simulink model "ITsystemThesis"  (R2025a)
settings: Solver=FixedStepAuto  StartTime=0.0  StopTime=0.55  FixedStep=50e-6  RelTol=1e-3
undefined symbols (not defined in the file): D1, Delta
libraries: spsSeriesRLCLoadLib x15, spsThreePhaseSeriesRLCLoadLib x12, spsPiSectionLineLib x12, spsThreePhasePISectionLineLib x11, spsThreePhaseVIMeasurementLib x7, spsThreePhaseTransformerTwoWindingsLib x6, spsSequenceAnalyzerLib x6, spsMultimeterLib x4, spsThreePhaseFaultLib x3, spsVoltageMeasurementLib x3, spsGroundLib x2, spsThreePhaseSourceLib x1
settings Model: Creator=baofengbaofeng  LastModifiedBy=baofeng
settings ModelReferenceCC: EnableRefExpFcnMdlSchedulingChecks=on
settings RTWCC: GPUComputeCapability=3.5  DLArmComputeVersion=19.05

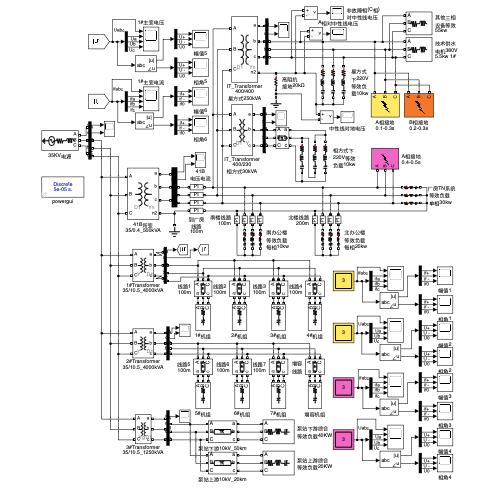
[thumbnail: Simulink's stored preview of the top-level diagram]
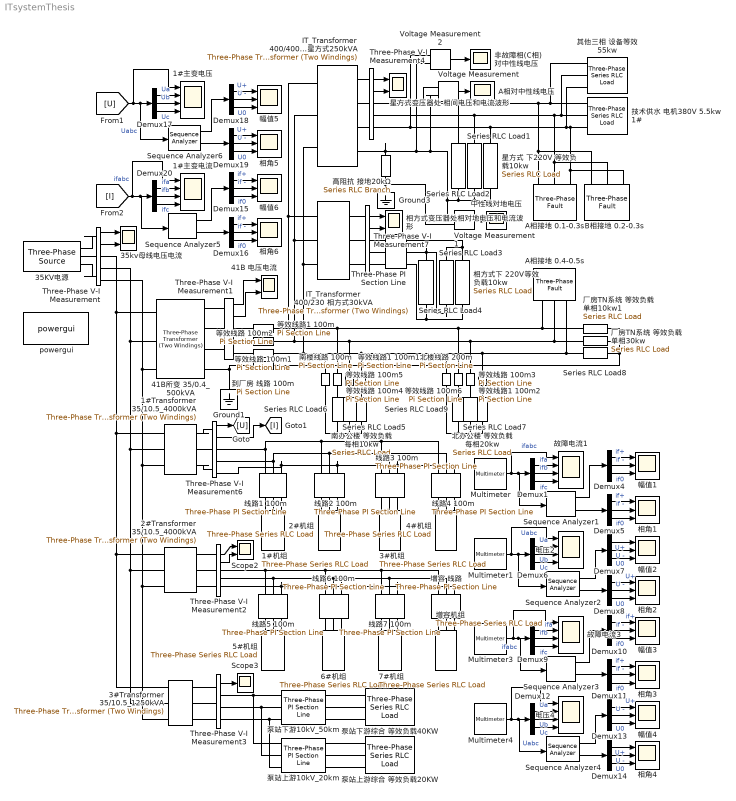
== system ITsystemThesis ==
  "    厂房TN系统 等效负载 单相10kw1" : spsSeriesRLCLoadLib/Series RLC Load  LConnTagsString=a  RConnTagsString=__new0  NominalVoltage=230  NominalFrequency=50  ActivePower=10e3  InductivePower=100  CapacitivePower=100  Setx0=off  InitialVoltage=0  SetiL0=off  InitialCurrent=0  Measurements=None  LoadType=constant Z
  "    厂房TN系统 等效负载 单相30kw" : spsSeriesRLCLoadLib/Series RLC Load  LConnTagsString=a  RConnTagsString=__new0  NominalVoltage=230  NominalFrequency=50  ActivePower=10e3  InductivePower=100  CapacitivePower=100  Setx0=off  InitialVoltage=0  SetiL0=off  InitialCurrent=0  Measurements=None  LoadType=constant Z
  1#Transformer 35/10.5_4000kVA : spsThreePhaseTransformerTwoWindingsLib/Three-Phase Transformer (Two Windings)  Winding1Connection=Y  Winding2Connection=Delta (D1)  CoreType=Three single-phase transformers  SetSaturation=off  Hysteresis=off  DataFile='hysteresis'  SetInitialFlux=off  Measurements=None  UNITS=pu  NominalPower=[4e6 , 50 ]  Winding1=[35000 0.01 0.049999]  Winding2=[10.5e3 0.01 0.05]  Rm=500  Lm=500  L0=0.5  Saturation=[0 0;0.0024 1.2;0.99998 1.52]  InitialFluxes=[ 0.8 , -0.8 , 0.7 ]  BreakLoop=off  DiscreteSolver=Trapezoidal iterative  DataType=off  TransfoNumber=1
  1#主变电压 : Scope  NumInputPorts=4
      settings: ActiveDisplayYMinimum=-10885.8844835699  ActiveDisplayYMaximum=10885.75905010345
  1#主变电流 : Scope  NumInputPorts=4
      settings: ActiveDisplayYMinimum=-290.20750490903231  ActiveDisplayYMaximum=290.20954287182195
  1#机组 : spsThreePhaseSeriesRLCLoadLib/Three-Phase Series RLC Load  LConnTagsString=A|B|C  Configuration=Delta  NominalVoltage=10e3  Vabc=[1e3 1e3 1e3]  Vabcp=[1e3 1e3 1e3]  NominalFrequency=50  UnbalancedPower=off  ActivePower=600e3  InductivePower=0  CapacitivePower=290e3  Pabc=[10e3 9e3 11e3]  QLabc=[100 90 110]  QCabc=[100 90 110]  Pabcp=[10e3 9e3 11e3]  QLabcp=[100 90 110]  QCabcp=[100 90 110]  Measurements=None  LoadType=constant PQ
  2#Transformer 35/10.5_4000kVA : spsThreePhaseTransformerTwoWindingsLib/Three-Phase Transformer (Two Windings)  Winding1Connection=Y  Winding2Connection=Delta (D1)  CoreType=Three single-phase transformers  SetSaturation=off  Hysteresis=off  DataFile='hysteresis'  SetInitialFlux=off  Measurements=None  UNITS=pu  NominalPower=[4e6 , 50 ]  Winding1=[35000 0.01 0.049999]  Winding2=[10.5e3 0.01 0.05]  Rm=500  Lm=500  L0=0.5  Saturation=[0 0;0.0024 1.2;0.99998 1.52]  InitialFluxes=[ 0.8 , -0.8 , 0.7 ]  BreakLoop=off  DiscreteSolver=Trapezoidal iterative  DataType=off  TransfoNumber=1
  2#机组 : spsThreePhaseSeriesRLCLoadLib/Three-Phase Series RLC Load  LConnTagsString=A|B|C  Configuration=Delta  NominalVoltage=10e3  Vabc=[1e3 1e3 1e3]  Vabcp=[1e3 1e3 1e3]  NominalFrequency=50  UnbalancedPower=off  ActivePower=600e3  InductivePower=0  CapacitivePower=290e3  Pabc=[10e3 9e3 11e3]  QLabc=[100 90 110]  QCabc=[100 90 110]  Pabcp=[10e3 9e3 11e3]  QLabcp=[100 90 110]  QCabcp=[100 90 110]  Measurements=None  LoadType=constant PQ
  3#Transformer 35/10.5_1250kVA : spsThreePhaseTransformerTwoWindingsLib/Three-Phase Transformer (Two Windings)  Winding1Connection=Yg  Winding2Connection=Delta (D1)  CoreType=Three single-phase transformers  SetSaturation=off  Hysteresis=off  DataFile='hysteresis'  SetInitialFlux=off  Measurements=None  UNITS=pu  NominalPower=[1250e3 , 50 ]  Winding1=[35000 0.01 0.049999]  Winding2=[10.5e3 0.01 0.05]  Rm=500  Lm=500  L0=0.5  Saturation=[0 0;0.0024 1.2;0.99998 1.52]  InitialFluxes=[ 0.8 , -0.8 , 0.7 ]  BreakLoop=off  DiscreteSolver=Trapezoidal iterative  DataType=off  TransfoNumber=1
  3#机组 : spsThreePhaseSeriesRLCLoadLib/Three-Phase Series RLC Load  LConnTagsString=A|B|C  Configuration=Delta  NominalVoltage=10e3  Vabc=[1e3 1e3 1e3]  Vabcp=[1e3 1e3 1e3]  NominalFrequency=50  UnbalancedPower=off  ActivePower=600e3  InductivePower=0  CapacitivePower=290e3  Pabc=[10e3 9e3 11e3]  QLabc=[100 90 110]  QCabc=[100 90 110]  Pabcp=[10e3 9e3 11e3]  QLabcp=[100 90 110]  QCabcp=[100 90 110]  Measurements=None  LoadType=constant PQ
  35KV电源 : spsThreePhaseSourceLib/Three-Phase Source  InternalConnection=Yg  VoltagePhases=off  Voltage=35e3  PhaseAngle=0  Voltage_phases=[25e3 25e3 25e3]/sqrt(3)  PhaseAngles_phases=[0 -120 +120]  Frequency=50  NonIdealSource=on  SpecifyImpedance=off  Resistance=0.1  Inductance=0.1e-3  ShortCircuitLevel=100e6  BaseVoltage=35e3  XRratio=7  BusType=swing  Pref=10e3  Qref=0  Prefabc=[10e3, 10e3, 10e3]  Qrefabc=[0, 0, 0]  Qmin=-inf  Qmax=inf
  35kv母线电压电流 : Scope  NumInputPorts=2
      settings: ActiveDisplayYMinimum=-35706.846494267083  ActiveDisplayYMaximum=35707.041687054967  DataLoggingVariableName=ScopeData6
  4#机组 : spsThreePhaseSeriesRLCLoadLib/Three-Phase Series RLC Load  LConnTagsString=A|B|C  Configuration=Delta  NominalVoltage=10e3  Vabc=[1e3 1e3 1e3]  Vabcp=[1e3 1e3 1e3]  NominalFrequency=50  UnbalancedPower=off  ActivePower=600e3  InductivePower=0  CapacitivePower=290e3  Pabc=[10e3 9e3 11e3]  QLabc=[100 90 110]  QCabc=[100 90 110]  Pabcp=[10e3 9e3 11e3]  QLabcp=[100 90 110]  QCabcp=[100 90 110]  Measurements=None  LoadType=constant PQ
  41B 电压电流 : Scope  NumInputPorts=2
      settings: ActiveDisplayYMinimum=-693.505234778138  ActiveDisplayYMaximum=693.42851734573628  DataLoggingVariableName=ScopeData2
  41B所变 35/0.4_500kVA : spsThreePhaseTransformerTwoWindingsLib/Three-Phase Transformer (Two Windings)  Winding1Connection=Delta (D1)  Winding2Connection=Yn  CoreType=Three single-phase transformers  SetSaturation=off  Hysteresis=off  DataFile='hysteresis'  SetInitialFlux=off  Measurements=None  UNITS=pu  NominalPower=[500e3 , 50 ]  Winding1=[35000 0.01 0.049999]  Winding2=[400 0.01 0.05]  Rm=500  Lm=499.99  L0=0.5  Saturation=[0 0;0.0024 1.2;0.99998 1.52]  InitialFluxes=[ 0.8 , -0.8 , 0.7 ]  BreakLoop=off  DiscreteSolver=Trapezoidal iterative  DataType=off  TransfoNumber=1
  5#机组 : spsThreePhaseSeriesRLCLoadLib/Three-Phase Series RLC Load  LConnTagsString=A|B|C  Configuration=Y (floating)  NominalVoltage=10e3  Vabc=[1e3 1e3 1e3]  Vabcp=[1e3 1e3 1e3]  NominalFrequency=50  UnbalancedPower=off  ActivePower=600e3  InductivePower=0  CapacitivePower=290e3  Pabc=[10e3 9e3 11e3]  QLabc=[100 90 110]  QCabc=[100 90 110]  Pabcp=[10e3 9e3 11e3]  QLabcp=[100 90 110]  QCabcp=[100 90 110]  Measurements=None  LoadType=constant PQ
  6#机组 : spsThreePhaseSeriesRLCLoadLib/Three-Phase Series RLC Load  LConnTagsString=A|B|C  Configuration=Y (floating)  NominalVoltage=10e3  Vabc=[1e3 1e3 1e3]  Vabcp=[1e3 1e3 1e3]  NominalFrequency=50  UnbalancedPower=off  ActivePower=600e3  InductivePower=0  CapacitivePower=290e3  Pabc=[10e3 9e3 11e3]  QLabc=[100 90 110]  QCabc=[100 90 110]  Pabcp=[10e3 9e3 11e3]  QLabcp=[100 90 110]  QCabcp=[100 90 110]  Measurements=None  LoadType=constant PQ
  7#机组 : spsThreePhaseSeriesRLCLoadLib/Three-Phase Series RLC Load  LConnTagsString=A|B|C  Configuration=Y (floating)  NominalVoltage=10e3  Vabc=[1e3 1e3 1e3]  Vabcp=[1e3 1e3 1e3]  NominalFrequency=50  UnbalancedPower=off  ActivePower=600e3  InductivePower=0  CapacitivePower=290e3  Pabc=[10e3 9e3 11e3]  QLabc=[100 90 110]  QCabc=[100 90 110]  Pabcp=[10e3 9e3 11e3]  QLabcp=[100 90 110]  QCabcp=[100 90 110]  Measurements=None  LoadType=constant PQ
  A相对中性线电压 : Scope
      settings: ActiveDisplayYMinimum=-1  ActiveDisplayYMaximum=1  DataLoggingVariableName=ScopeData7
  A相接地 0.1-0.3s : spsThreePhaseFaultLib/Three-Phase Fault  InitialStates=0  FaultA=on  FaultB=off  FaultC=off  GroundFault=on  SwitchTimes="[5/50  15/50]"  External=off  SwitchStatus=NaN  FaultResistance=0.001  GroundResistance=0.01  SnubberResistance=20e3  SnubberCapacitance=1  Measurements=Fault voltages and currents
  A相接地 0.4-0.5s : spsThreePhaseFaultLib/Three-Phase Fault  InitialStates=0  FaultA=on  FaultB=off  FaultC=off  GroundFault=on  SwitchTimes="[20/50  25/50]"  External=off  SwitchStatus=NaN  FaultResistance=0.001  GroundResistance=0.01  SnubberResistance=1e3  SnubberCapacitance=inf  Measurements=Fault voltages and currents
  B相接地 0.2-0.3s : spsThreePhaseFaultLib/Three-Phase Fault  InitialStates=0  FaultA=off  FaultB=on  FaultC=off  GroundFault=on  SwitchTimes="[10/50  15/50]"  External=off  SwitchStatus=NaN  FaultResistance=0.001  GroundResistance=0.01  SnubberResistance=20e3  SnubberCapacitance=inf  Measurements=Fault voltages and currents
  Demux{1,4..20} (18 alike) : Demux  Outputs=3
  Ground1 : spsGroundLib/Ground  LConnTagsString=a
  Ground3 : spsGroundLib/Ground  LConnTagsString=a
  IT_Transformer 400/230 相方式30kVA : spsThreePhaseTransformerTwoWindingsLib/Three-Phase Transformer (Two Windings)  Winding1Connection=Delta (D1)  Winding2Connection=Y  CoreType=Three single-phase transformers  SetSaturation=off  Hysteresis=off  DataFile='hysteresis'  SetInitialFlux=off  Measurements=None  UNITS=pu  NominalPower=[30e3 , 50 ]  Winding1=[400, 0.002 , 0.08 ]  Winding2=[230, 0.002 , 0.08 ]  Rm=500  Lm=500  L0=0.5  Saturation=[ 0,0 ; 0.0024,1.2 ; 1.0,1.52 ]  InitialFluxes=[ 0.8 , -0.8 , 0.7 ]  BreakLoop=off  DiscreteSolver=Trapezoidal iterative  DataType=off  TransfoNumber=1
  IT_Transformer 400/400 星方式250kVA : spsThreePhaseTransformerTwoWindingsLib/Three-Phase Transformer (Two Windings)  Winding1Connection=Delta (D1)  Winding2Connection=Yn  CoreType=Three single-phase transformers  SetSaturation=off  Hysteresis=off  DataFile='hysteresis'  SetInitialFlux=off  Measurements=None  UNITS=pu  NominalPower=[ 250e3 , 50 ]  Winding1=[ 400 , 0.002 , 0.08 ]  Winding2=[ 400 , 0.002 , 0.08 ]  Rm=500  Lm=500  L0=0.5  Saturation=[ 0,0 ; 0.0024,1.2 ; 1.0,1.52 ]  InitialFluxes=[ 0.8 , -0.8 , 0.7 ]  BreakLoop=off  DiscreteSolver=Trapezoidal iterative  DataType=off  TransfoNumber=1
  Multimeter : spsMultimeterLib/Multimeter  L=12  sel=[7 8 9]  yselected={}  Gain=[1 1 1]  OutputType=Complex  PlotAtSimulationStop=off  PhasorSimulation=off
  Multimeter1 : spsMultimeterLib/Multimeter  L=12  sel=[1 2 3]  yselected={}  Gain=[1 1 1]  OutputType=Complex  PlotAtSimulationStop=off  PhasorSimulation=off
  Multimeter3 : spsMultimeterLib/Multimeter  L=12  sel=[10 11 12]  yselected={}  Gain=[1 1 1]  OutputType=Complex  PlotAtSimulationStop=off  PhasorSimulation=off
  Multimeter4 : spsMultimeterLib/Multimeter  L=12  sel=[4 5 6]  yselected={}  Gain=[1 1 1]  OutputType=Complex  PlotAtSimulationStop=off  PhasorSimulation=off
  Scope2 : Scope  NumInputPorts=2
      settings: ActiveDisplayYMinimum=-10885.884483600445  ActiveDisplayYMaximum=10885.759050087665  DataLoggingVariableName=ScopeData4
  Scope3 : Scope
      settings: ActiveDisplayYMinimum=-10727.159391884898  ActiveDisplayYMaximum=10726.597579018544  DataLoggingVariableName=ScopeData5
  Sequence Analyzer{1..6} (6 alike) : spsSequenceAnalyzerLib/Sequence Analyzer  Freq=50  n=1  seq=Positive Negative Zero  InInit=[1, 0]  Ts=0
      settings: LibrarySourceBlock=sps_lib/Sensors and Measurements/Sequence Analyzer
  Series RLC Load{1..6,8} (7 alike) : spsSeriesRLCLoadLib/Series RLC Load  LConnTagsString=a  RConnTagsString=__new0  NominalVoltage=230  NominalFrequency=50  ActivePower=10e3  InductivePower=100  CapacitivePower=100  Setx0=off  InitialVoltage=0  SetiL0=off  InitialCurrent=0  Measurements=None  LoadType=constant Z
  Series RLC Load7 : spsSeriesRLCLoadLib/Series RLC Load  LConnTagsString=a  RConnTagsString=__new0  NominalVoltage=230  NominalFrequency=50  ActivePower=20e3  InductivePower=100  CapacitivePower=100  Setx0=off  InitialVoltage=0  SetiL0=off  InitialCurrent=0  Measurements=None  LoadType=constant Z
  Series RLC Load9 : spsSeriesRLCLoadLib/Series RLC Load  LConnTagsString=a  RConnTagsString=__new0  NominalVoltage=230  NominalFrequency=50  ActivePower=20e3  InductivePower=100  CapacitivePower=100  Setx0=off  InitialVoltage=0  SetiL0=off  InitialCurrent=0  Measurements=None  LoadType=constant Z
  Three-Phase PI Section Line : spsThreePhasePISectionLineLib/Three-Phase PI Section Line  LConnTagsString=a|b|c  RConnTagsString=A|B|C  Length=100  Frequency=60  Resistances=[ 0.01273 0.3864]  Inductances="[ 0.9337e-3  4.1264e-3]"  Capacitances=[12.74e-9 7.751e-9]
  Three-Phase V-I Measurement{,2,6..7} (4 alike) : spsThreePhaseVIMeasurementLib/Three-Phase V-I Measurement  VoltageMeasurement=phase-to-ground  SetLabelV=off  LabelV=Vabc  Vpu=off  VpuLL=off  CurrentMeasurement=yes  SetLabelI=off  LabelI=Iabc  Ipu=off  Pbase=100e6  Vbase=500e3  OutputType=Complex  PhasorSimulation=off  PSBequivalent=0
  Three-Phase V-I Measurement1 : spsThreePhaseVIMeasurementLib/Three-Phase V-I Measurement  VoltageMeasurement=phase-to-phase  SetLabelV=off  LabelV=Vabc  Vpu=off  VpuLL=off  CurrentMeasurement=yes  SetLabelI=off  LabelI=Iabc  Ipu=off  Pbase=100e6  Vbase=500e3  OutputType=Complex  PhasorSimulation=off  PSBequivalent=0
  Three-Phase V-I Measurement3 : spsThreePhaseVIMeasurementLib/Three-Phase V-I Measurement  VoltageMeasurement=phase-to-ground  SetLabelV=off  LabelV=Vabc  Vpu=off  VpuLL=off  CurrentMeasurement=no  SetLabelI=off  LabelI=Iabc  Ipu=off  Pbase=100e6  Vbase=500e3  OutputType=Complex  PhasorSimulation=off  PSBequivalent=0
  Three-Phase V-I Measurement4 : spsThreePhaseVIMeasurementLib/Three-Phase V-I Measurement  VoltageMeasurement=phase-to-phase  SetLabelV=off  LabelV=Vabc  Vpu=off  VpuLL=off  CurrentMeasurement=yes  SetLabelI=off  LabelI=Iabc  Ipu=off  Pbase=100e6  Vbase=500e3  OutputType=Complex  PhasorSimulation=off  PSBequivalent=0
  Voltage Measurement : spsVoltageMeasurementLib/Voltage Measurement  PhasorSimulation=off  OutputType=Complex  PSBequivalent=0
  Voltage Measurement1 : spsVoltageMeasurementLib/Voltage Measurement  PhasorSimulation=off  OutputType=Complex  PSBequivalent=0
  Voltage Measurement2 : spsVoltageMeasurementLib/Voltage Measurement  PhasorSimulation=off  OutputType=Complex  PSBequivalent=0
  powergui : spspowerguiLib/powergui  Priority=1  SimulationMode=Discrete  SampleTime=50e-6  frequency=50  Iterations=50  frequencyindice=50  Pbase=100e6  ErrMax=1e-4  UnitsV=kV  UnitsW=MW  buscounter=0  FunctionMessages=off  echomessages=off  EnableUseOfTLC=off  CurrentSourceSwitches=off  DisableSnubberDevices=off  DisableRonSwitches=off  DisableVfSwitches=off  DisplayEquations=off  AutomaticDiscreteSolvers=off  SolverType=Tustin/Backward Euler (TBE)  Interpol=off  ExternalGateDelay=off  methode=off  Ts=100  x0status=blocks  SPID=on  SwTol=0  HookPort=off  NonlinearTolerance=1e-4  nMaxIteration=100  ContinueOnMaxIteration=off  RestoreLinks=warning  ResistiveCurrentMeasurement=off  Frange=[0:2:500]  Ylog=off  Xlog=on  ShowGrid=off  save=off  variable=ZData  structure=0  ZoomFFT=off  StartTime=0.0  cycles=1  DisplayStyle=1  fundamental=60  FreqAxis=off  MaxFrequency=1000  frequencyindicesteady=1  RmsSteady=1  display=off
  中性线对地电压 : Scope
      settings: ActiveDisplayYMinimum=-386.53820546977795  ActiveDisplayYMaximum=386.53827874690307  DataLoggingVariableName=ScopeData8
  其他三相 设备等效 55kw : spsThreePhaseSeriesRLCLoadLib/Three-Phase Series RLC Load  LConnTagsString=A|B|C  Configuration=Y (floating)  NominalVoltage=380  Vabc=[1e3 1e3 1e3]  Vabcp=[1e3 1e3 1e3]  NominalFrequency=50  UnbalancedPower=off  ActivePower=55e3  InductivePower=27.5e3  CapacitivePower=0  Pabc=[10e3 9e3 11e3]  QLabc=[100 90 110]  QCabc=[100 90 110]  Pabcp=[10e3 9e3 11e3]  QLabcp=[100 90 110]  QCabcp=[100 90 110]  Measurements=None  LoadType=constant Z
  到厂房 线路 100m : spsPiSectionLineLib/Pi Section Line  LConnTagsString=1  RConnTagsString=1  Phases=1  PiSections=1  Length=0.1  Frequency=50  Resistance=0.01273  Inductance=0.9337e-3  Capacitance=12.74e-9  SpecifyConductance=off  Conductance=0  Measurements=None  Measurements2=None
      settings: LibrarySourceBlock=sps_lib/Power Grid Elements/Pi Section Line
  北办公楼 等效负载 每相20kw : spsSeriesRLCLoadLib/Series RLC Load  LConnTagsString=a  RConnTagsString=__new0  NominalVoltage=230  NominalFrequency=50  ActivePower=20e3  InductivePower=100  CapacitivePower=100  Setx0=off  InitialVoltage=0  SetiL0=off  InitialCurrent=0  Measurements=None  LoadType=constant Z
  北楼线路 200m : spsPiSectionLineLib/Pi Section Line  LConnTagsString=1  RConnTagsString=1  Phases=1  PiSections=1  Length=0.2  Frequency=50  Resistance=0.01273  Inductance=0.9337e-3  Capacitance=12.74e-9  SpecifyConductance=off  Conductance=0  Measurements=None  Measurements2=None
      settings: LibrarySourceBlock=sps_lib/Power Grid Elements/Pi Section Line
  南办公楼 等效负载 每相10kw : spsSeriesRLCLoadLib/Series RLC Load  LConnTagsString=a  RConnTagsString=__new0  NominalVoltage=230  NominalFrequency=50  ActivePower=10e3  InductivePower=100  CapacitivePower=100  Setx0=off  InitialVoltage=0  SetiL0=off  InitialCurrent=0  Measurements=None  LoadType=constant Z
  南楼线路 100m : spsPiSectionLineLib/Pi Section Line  LConnTagsString=1  RConnTagsString=1  Phases=1  PiSections=1  Length=0.1  Frequency=50  Resistance=0.01273  Inductance=0.9337e-3  Capacitance=12.74e-9  SpecifyConductance=off  Conductance=0  Measurements=None  Measurements2=None
      settings: LibrarySourceBlock=sps_lib/Power Grid Elements/Pi Section Line
  增容 线路 : spsThreePhasePISectionLineLib/Three-Phase PI Section Line  LConnTagsString=a|b|c  RConnTagsString=A|B|C  Length=0.1  Frequency=50  Resistances=[ 0.01273 0.3864]  Inductances="[ 0.9337e-3  4.1264e-3]"  Capacitances=[12.74e-9 7.751e-9]
  增容机组 : spsThreePhaseSeriesRLCLoadLib/Three-Phase Series RLC Load  LConnTagsString=A|B|C  Configuration=Y (floating)  NominalVoltage=10e3  Vabc=[1e3 1e3 1e3]  Vabcp=[1e3 1e3 1e3]  NominalFrequency=50  UnbalancedPower=off  ActivePower=600e3  InductivePower=0  CapacitivePower=290e3  Pabc=[10e3 9e3 11e3]  QLabc=[100 90 110]  QCabc=[100 90 110]  Pabcp=[10e3 9e3 11e3]  QLabcp=[100 90 110]  QCabcp=[100 90 110]  Measurements=None  LoadType=constant PQ
  幅值{1..6} (6 alike) : Scope  NumInputPorts=3
      幅值1 settings: ActiveDisplayYMinimum=-0.00269711612383589  ActiveDisplayYMaximum=0.024274045114523017  DataLoggingVariableName=ScopeData11
      幅值2 settings: ActiveDisplayYMinimum=-37.543097825269918  ActiveDisplayYMaximum=347.88788042742931  DataLoggingVariableName=ScopeData14
      幅值3 settings: ActiveDisplayYMinimum=-237.57858107654377  ActiveDisplayYMaximum=2138.2072296888946  DataLoggingVariableName=ScopeData19
      幅值4 settings: ActiveDisplayYMinimum=-39.338118269801356  ActiveDisplayYMaximum=364.04306442821229  DataLoggingVariableName=ScopeData20
      幅值5 settings: ActiveDisplayYMinimum=-1087.411711387326  ActiveDisplayYMaximum=9796.7054024859353  DataLoggingVariableName=ScopeData24
      幅值6 settings: ActiveDisplayYMinimum=-27.894504137772689  ActiveDisplayYMaximum=261.05053723995428  DataLoggingVariableName=ScopeData23
  技术供水 电机380V 5.5kw 1# : spsThreePhaseSeriesRLCLoadLib/Three-Phase Series RLC Load  LConnTagsString=A|B|C  Configuration=Y (floating)  NominalVoltage=380  Vabc=[1e3 1e3 1e3]  Vabcp=[1e3 1e3 1e3]  NominalFrequency=50  UnbalancedPower=off  ActivePower=5.5e3  InductivePower=2.75e3  CapacitivePower=0  Pabc=[10e3 9e3 11e3]  QLabc=[100 90 110]  QCabc=[100 90 110]  Pabcp=[10e3 9e3 11e3]  QLabcp=[100 90 110]  QCabcp=[100 90 110]  Measurements=None  LoadType=constant Z
  故障电流1 : Scope  NumInputPorts=4
      settings: ActiveDisplayYMinimum=-2115.6411271895017  ActiveDisplayYMaximum=2117.5918585380573  DataLoggingVariableName=ScopeData3
  故障电流3 : Scope  NumInputPorts=4
      settings: ActiveDisplayYMinimum=-6472.8025751599744  ActiveDisplayYMaximum=8249.2362367472233  DataLoggingVariableName=ScopeData18
  星方式 下220V 等效负 载10kw : spsSeriesRLCLoadLib/Series RLC Load  LConnTagsString=a  RConnTagsString=__new0  NominalVoltage=230  NominalFrequency=50  ActivePower=10e3  InductivePower=100  CapacitivePower=100  Setx0=off  InitialVoltage=0  SetiL0=off  InitialCurrent=0  Measurements=None  LoadType=constant Z
  星方式变压器处 相间电压和电流波形 : Scope  NumInputPorts=2
      settings: ActiveDisplayYMinimum=-670.32665640027585  ActiveDisplayYMaximum=669.92281587607806  DataLoggingVariableName=ScopeData15
  泵站上游10kV_20km : spsThreePhasePISectionLineLib/Three-Phase PI Section Line  LConnTagsString=a|b|c  RConnTagsString=A|B|C  Length=20  Frequency=50  Resistances=[ 0.01273 0.3864]  Inductances="[ 0.9337e-3  4.1264e-3]"  Capacitances=[12.74e-9 7.751e-9]
  泵站上游综合 等效负载20KW : spsThreePhaseSeriesRLCLoadLib/Three-Phase Series RLC Load  LConnTagsString=A|B|C  Configuration=Y (floating)  NominalVoltage=10e3  Vabc=[1e3 1e3 1e3]  Vabcp=[1e3 1e3 1e3]  NominalFrequency=50  UnbalancedPower=off  ActivePower=20e3  InductivePower=100  CapacitivePower=100  Pabc=[10e3 9e3 11e3]  QLabc=[100 90 110]  QCabc=[100 90 110]  Pabcp=[10e3 9e3 11e3]  QLabcp=[100 90 110]  QCabcp=[100 90 110]  Measurements=None  LoadType=constant Z
  泵站下游10kV_50km : spsThreePhasePISectionLineLib/Three-Phase PI Section Line  LConnTagsString=a|b|c  RConnTagsString=A|B|C  Length=50  Frequency=50  Resistances=[ 0.01273 0.3864]  Inductances="[ 0.9337e-3  4.1264e-3]"  Capacitances=[12.74e-9 7.751e-9]
  泵站下游综合 等效负载40KW : spsThreePhaseSeriesRLCLoadLib/Three-Phase Series RLC Load  LConnTagsString=A|B|C  Configuration=Y (floating)  NominalVoltage=10e3  Vabc=[1e3 1e3 1e3]  Vabcp=[1e3 1e3 1e3]  NominalFrequency=50  UnbalancedPower=off  ActivePower=40e3  InductivePower=100  CapacitivePower=100  Pabc=[10e3 9e3 11e3]  QLabc=[100 90 110]  QCabc=[100 90 110]  Pabcp=[10e3 9e3 11e3]  QLabcp=[100 90 110]  QCabcp=[100 90 110]  Measurements=None  LoadType=constant Z
  电压2 : Scope  NumInputPorts=4
      settings: ActiveDisplayYMinimum=-669.7122622202794  ActiveDisplayYMaximum=669.712217692271  DataLoggingVariableName=ScopeData12
  电压4 : Scope  NumInputPorts=4
      settings: ActiveDisplayYMinimum=-475.45137271071371  ActiveDisplayYMaximum=457.036637182715  DataLoggingVariableName=ScopeData17
  相方式下 220V等效 负载10kw : spsSeriesRLCLoadLib/Series RLC Load  LConnTagsString=a  RConnTagsString=__new0  NominalVoltage=230  NominalFrequency=50  ActivePower=10e3  InductivePower=100  CapacitivePower=100  Setx0=off  InitialVoltage=0  SetiL0=off  InitialCurrent=0  Measurements=None  LoadType=constant Z
  相方式变压器处相对地电压和电流波形 : Scope  NumInputPorts=2
      settings: ActiveDisplayYMinimum=-229.68543143110043  ActiveDisplayYMaximum=227.02248165488766  DataLoggingVariableName=ScopeData16
  相角{1..6} (6 alike) : Scope  NumInputPorts=3
      相角1 settings: ActiveDisplayYMinimum=-1  ActiveDisplayYMaximum=1  DataLoggingVariableName=ScopeData10
      相角2 settings: ActiveDisplayYMinimum=-7.0496414728403192  ActiveDisplayYMaximum=63.446773255562888  DataLoggingVariableName=ScopeData13
      相角3 settings: ActiveDisplayYMinimum=-160.42500077107547  ActiveDisplayYMaximum=116.32499922893246  DataLoggingVariableName=ScopeData21
      相角4 settings: ActiveDisplayYMinimum=-3.4641360988234386  ActiveDisplayYMaximum=31.177224889410954  DataLoggingVariableName=ScopeData22
      相角5 settings: ActiveDisplayYMinimum=-39.040360895201125  ActiveDisplayYMaximum=4.3378178772445688  DataLoggingVariableName=ScopeData26
      相角6 settings: ActiveDisplayYMinimum=-1  ActiveDisplayYMaximum=1  DataLoggingVariableName=ScopeData25
  等效线路 100m{1..2,4..5} (4 alike) : spsPiSectionLineLib/Pi Section Line  LConnTagsString=1  RConnTagsString=1  Phases=1  PiSections=1  Length=0.1  Frequency=50  Resistance=0.01273  Inductance=0.9337e-3  Capacitance=12.74e-9  SpecifyConductance=off  Conductance=0  Measurements=None  Measurements2=None
      settings: LibrarySourceBlock=sps_lib/Power Grid Elements/Pi Section Line
  等效线路 100m3 : spsPiSectionLineLib/Pi Section Line  LConnTagsString=1  RConnTagsString=1  Phases=1  PiSections=1  Length=0.2  Frequency=50  Resistance=0.01273  Inductance=0.9337e-3  Capacitance=12.74e-9  SpecifyConductance=off  Conductance=0  Measurements=None  Measurements2=None
      settings: LibrarySourceBlock=sps_lib/Power Grid Elements/Pi Section Line
  等效线路 100m6 : spsPiSectionLineLib/Pi Section Line  LConnTagsString=1  RConnTagsString=1  Phases=1  PiSections=1  Length=0.2  Frequency=50  Resistance=0.01273  Inductance=0.9337e-3  Capacitance=12.74e-9  SpecifyConductance=off  Conductance=0  Measurements=None  Measurements2=None
      settings: LibrarySourceBlock=sps_lib/Power Grid Elements/Pi Section Line
  等效线路1 100m : spsPiSectionLineLib/Pi Section Line  LConnTagsString=1  RConnTagsString=1  Phases=1  PiSections=1  Length=0.1  Frequency=50  Resistance=0.01273  Inductance=0.9337e-3  Capacitance=12.74e-9  SpecifyConductance=off  Conductance=0  Measurements=None  Measurements2=None
      settings: LibrarySourceBlock=sps_lib/Power Grid Elements/Pi Section Line
  等效线路1 100m1 : spsPiSectionLineLib/Pi Section Line  LConnTagsString=1  RConnTagsString=1  Phases=1  PiSections=1  Length=0.1  Frequency=50  Resistance=0.01273  Inductance=0.9337e-3  Capacitance=12.74e-9  SpecifyConductance=off  Conductance=0  Measurements=None  Measurements2=None
      settings: LibrarySourceBlock=sps_lib/Power Grid Elements/Pi Section Line
  等效线路1 100m2 : spsPiSectionLineLib/Pi Section Line  LConnTagsString=1  RConnTagsString=1  Phases=1  PiSections=1  Length=0.2  Frequency=50  Resistance=0.01273  Inductance=0.9337e-3  Capacitance=12.74e-9  SpecifyConductance=off  Conductance=0  Measurements=None  Measurements2=None
      settings: LibrarySourceBlock=sps_lib/Power Grid Elements/Pi Section Line
  线路1 100m : spsThreePhasePISectionLineLib/Three-Phase PI Section Line  LConnTagsString=a|b|c  RConnTagsString=A|B|C  Length=0.1  Frequency=50  Resistances=[ 0.01273 0.3864]  Inductances="[ 0.9337e-3  4.1264e-3]"  Capacitances=[12.74e-9 7.751e-9]
  线路2 100m : spsThreePhasePISectionLineLib/Three-Phase PI Section Line  LConnTagsString=a|b|c  RConnTagsString=A|B|C  Length=0.1  Frequency=50  Resistances=[ 0.01273 0.3864]  Inductances="[ 0.9337e-3  4.1264e-3]"  Capacitances=[12.74e-9 7.751e-9]
  线路3 100m : spsThreePhasePISectionLineLib/Three-Phase PI Section Line  LConnTagsString=a|b|c  RConnTagsString=A|B|C  Length=0.1  Frequency=50  Resistances=[ 0.01273 0.3864]  Inductances="[ 0.9337e-3  4.1264e-3]"  Capacitances=[12.74e-9 7.751e-9]
  线路4 100m : spsThreePhasePISectionLineLib/Three-Phase PI Section Line  LConnTagsString=a|b|c  RConnTagsString=A|B|C  Length=0.1  Frequency=50  Resistances=[ 0.01273 0.3864]  Inductances="[ 0.9337e-3  4.1264e-3]"  Capacitances=[12.74e-9 7.751e-9]
  线路5 100m : spsThreePhasePISectionLineLib/Three-Phase PI Section Line  LConnTagsString=a|b|c  RConnTagsString=A|B|C  Length=0.1  Frequency=50  Resistances=[ 0.01273 0.3864]  Inductances="[ 0.9337e-3  4.1264e-3]"  Capacitances=[12.74e-9 7.751e-9]
  线路6 100m : spsThreePhasePISectionLineLib/Three-Phase PI Section Line  LConnTagsString=a|b|c  RConnTagsString=A|B|C  Length=0.1  Frequency=50  Resistances=[ 0.01273 0.3864]  Inductances="[ 0.9337e-3  4.1264e-3]"  Capacitances=[12.74e-9 7.751e-9]
  线路7 100m : spsThreePhasePISectionLineLib/Three-Phase PI Section Line  LConnTagsString=a|b|c  RConnTagsString=A|B|C  Length=0.1  Frequency=50  Resistances=[ 0.01273 0.3864]  Inductances="[ 0.9337e-3  4.1264e-3]"  Capacitances=[12.74e-9 7.751e-9]
  非故障相(C相) 对中性线电压 : Scope
      settings: ActiveDisplayYMinimum=-1  ActiveDisplayYMaximum=1  DataLoggingVariableName=ScopeData9
  高阻抗 接地20kΩ : spsSeriesRLCBranchLib/Series RLC Branch  LConnTagsString=__new0  RConnTagsString=__new0  BranchType=R  Resistance=20000  Inductance=0  SetiL0=off  InitialCurrent=0  Capacitance=0  Setx0=off  InitialVoltage=0  Measurements=None
  wires:
  Three-Phase V-I Measurement6/1 -> [U]
  Three-Phase V-I Measurement2/1 -> Scope2/1
  Three-Phase V-I Measurement/1 -> 35kv母线电压电流/1
  Three-Phase V-I Measurement3/1 -> Scope3/1
  Three-Phase V-I Measurement/2 -> 35kv母线电压电流/2
  Three-Phase V-I Measurement1/2 -> 41B 电压电流/2
  Three-Phase V-I Measurement2/2 -> Scope2/2
  Three-Phase V-I Measurement1/1 -> 41B 电压电流/1
  Demux5/3 -> 相角1/3  "if0"
  Demux1/3 -> 故障电流1/4  "ifc"
  Multimeter/1 -> Sequence Analyzer1/1, Demux1/1, 故障电流1/1  "ifabc"
  Demux5/1 -> 相角1/1  "if+"
  Demux5/2 -> 相角1/2  "if -"
  Demux1/1 -> 故障电流1/2  "ifa"
  Demux4/3 -> 幅值1/3  "if0"
  Demux1/2 -> 故障电流1/3  "ifb"
  Demux4/1 -> 幅值1/1  "if+"
  Demux4/2 -> 幅值1/2  "if -"
  Sequence Analyzer1/2 -> Demux5/1
  Sequence Analyzer1/1 -> Demux4/1
  Demux7/3 -> 幅值2/3  "U0"
  Demux8/2 -> 相角2/2  "U -"
  Demux6/2 -> 电压2/3  "Ub"
  Demux6/3 -> 电压2/4  "Uc"
  Sequence Analyzer2/2 -> Demux8/1
  Demux7/1 -> 幅值2/1  "U+"
  Demux8/3 -> 相角2/3  "U0"
  Demux8/1 -> 相角2/1  "U+"
  Demux7/2 -> 幅值2/2  "U -"
  Multimeter1/1 -> 电压2/1, Demux6/1, Sequence Analyzer2/1  "Uabc"
  Sequence Analyzer2/1 -> Demux7/1
  Three-Phase V-I Measurement4/1 -> 星方式变压器处 相间电压和电流波形/1
  Three-Phase V-I Measurement4/2 -> 星方式变压器处 相间电压和电流波形/2
  Three-Phase V-I Measurement7/1 -> 相方式变压器处相对地电压和电流波形/1
  Three-Phase V-I Measurement7/2 -> 相方式变压器处相对地电压和电流波形/2
  Demux6/1 -> 电压2/2  "Ua"
  Demux12/1 -> 电压4/2  "Ua"
  Sequence Analyzer4/1 -> Demux13/1
  Multimeter4/1 -> Sequence Analyzer4/1, Demux12/1, 电压4/1  "Uabc"
  Demux13/2 -> 幅值4/2  "U -"
  Demux14/1 -> 相角4/1  "U+"
  Demux14/3 -> 相角4/3  "U0"
  Demux13/1 -> 幅值4/1  "U+"
  Sequence Analyzer4/2 -> Demux14/1
  Demux12/3 -> 电压4/4  "Uc"
  Demux12/2 -> 电压4/3  "Ub"
  Demux14/2 -> 相角4/2  "U -"
  Demux13/3 -> 幅值4/3  "U0"
  Sequence Analyzer3/1 -> Demux10/1
  Sequence Analyzer3/2 -> Demux11/1
  Demux10/2 -> 幅值3/2  "if -"
  Demux10/1 -> 幅值3/1  "if+"
  Demux9/2 -> 故障电流3/3  "ifb"
  Demux10/3 -> 幅值3/3  "if0"
  Demux9/1 -> 故障电流3/2  "ifa"
  Demux11/2 -> 相角3/2  "if -"
  Demux11/1 -> 相角3/1  "if+"
  Multimeter3/1 -> Sequence Analyzer3/1, Demux9/1, 故障电流3/1  "ifabc"
  Demux9/3 -> 故障电流3/4  "ifc"
  Demux11/3 -> 相角3/3  "if0"
  Demux16/2 -> 相角6/2  "if -"
  Demux16/1 -> 相角6/1  "if+"
  Demux18/3 -> 幅值5/3  "U0"
  Sequence Analyzer5/2 -> Demux16/1
  Demux19/3 -> 相角5/3  "U0"
  Demux18/2 -> 幅值5/2  "U -"
  [U] -> 1#主变电压/1, Sequence Analyzer6/1, Demux17/1  "Uabc"
  [I] -> 1#主变电流/1, Demux20/1, Sequence Analyzer5/1  "ifabc"
  Demux17/1 -> 1#主变电压/2  "Ua"
  Demux17/3 -> 1#主变电压/4  "Uc"
  Demux18/1 -> 幅值5/1  "U+"
  Demux20/2 -> 1#主变电流/3  "ifb"
  Demux19/1 -> 相角5/1  "U+"
  Sequence Analyzer6/1 -> Demux18/1
  Demux20/3 -> 1#主变电流/4  "ifc"
  Sequence Analyzer5/1 -> Demux15/1
  Demux15/3 -> 幅值6/3  "if0"
  Demux15/2 -> 幅值6/2  "if -"
  Demux17/2 -> 1#主变电压/3  "Ub"
  Demux15/1 -> 幅值6/1  "if+"
  Sequence Analyzer6/2 -> Demux19/1
  Demux19/2 -> 相角5/2  "U -"
  Demux20/1 -> 1#主变电流/2  "ifa"
  Demux16/3 -> 相角6/3  "if0"
  Three-Phase V-I Measurement6/2 -> [I]
  Voltage Measurement/1 -> A相对中性线电压/1
  Voltage Measurement1/1 -> 中性线对地电压/1
  Voltage Measurement2/1 -> 非故障相(C相) 对中性线电压/1
  connections:
  Three-Phase V-I Measurement/LConn2 -- 35KV电源/RConn2
  Three-Phase V-I Measurement/LConn3 -- 35KV电源/RConn3
  Three-Phase V-I Measurement/LConn1 -- 35KV电源/RConn1
  Three-Phase V-I Measurement/RConn1 -- 3#Transformer 35/10.5_1250kVA/LConn1 -- 2#Transformer 35/10.5_4000kVA/LConn1 -- 1#Transformer 35/10.5_4000kVA/LConn1 -- 41B所变 35/0.4_500kVA/LConn1
  Three-Phase V-I Measurement/RConn2 -- 3#Transformer 35/10.5_1250kVA/LConn2 -- 2#Transformer 35/10.5_4000kVA/LConn2 -- 1#Transformer 35/10.5_4000kVA/LConn2 -- 41B所变 35/0.4_500kVA/LConn2
  Three-Phase V-I Measurement/RConn3 -- 3#Transformer 35/10.5_1250kVA/LConn3 -- 2#Transformer 35/10.5_4000kVA/LConn3 -- 1#Transformer 35/10.5_4000kVA/LConn3 -- 41B所变 35/0.4_500kVA/LConn3
  Three-Phase V-I Measurement1/LConn1 -- 41B所变 35/0.4_500kVA/RConn1
  Three-Phase V-I Measurement1/LConn2 -- 41B所变 35/0.4_500kVA/RConn2
  Three-Phase V-I Measurement1/LConn3 -- 41B所变 35/0.4_500kVA/RConn3
  1#Transformer 35/10.5_4000kVA/RConn1 -- Three-Phase V-I Measurement6/LConn1
  1#Transformer 35/10.5_4000kVA/RConn2 -- Three-Phase V-I Measurement6/LConn2
  1#Transformer 35/10.5_4000kVA/RConn3 -- Three-Phase V-I Measurement6/LConn3
  3#Transformer 35/10.5_1250kVA/RConn1 -- Three-Phase V-I Measurement3/LConn1
  3#Transformer 35/10.5_1250kVA/RConn2 -- Three-Phase V-I Measurement3/LConn2
  3#Transformer 35/10.5_1250kVA/RConn3 -- Three-Phase V-I Measurement3/LConn3
  Three-Phase V-I Measurement2/RConn1 -- 线路7 100m/LConn1 -- 增容 线路/LConn1 -- 线路6 100m/LConn1 -- 线路5 100m/LConn1
  Three-Phase V-I Measurement2/RConn2 -- 线路7 100m/LConn2 -- 增容 线路/LConn2 -- 线路6 100m/LConn2 -- 线路5 100m/LConn2
  Three-Phase V-I Measurement2/RConn3 -- 线路5 100m/LConn3 -- 线路6 100m/LConn3 -- 线路7 100m/LConn3 -- 增容 线路/LConn3
  2#Transformer 35/10.5_4000kVA/RConn1 -- Three-Phase V-I Measurement2/LConn1
  2#Transformer 35/10.5_4000kVA/RConn2 -- Three-Phase V-I Measurement2/LConn2
  2#Transformer 35/10.5_4000kVA/RConn3 -- Three-Phase V-I Measurement2/LConn3
  Three-Phase V-I Measurement3/RConn1 -- 泵站上游10kV_20km/LConn1 -- 泵站下游10kV_50km/LConn1
  Three-Phase V-I Measurement3/RConn2 -- 泵站上游10kV_20km/LConn2 -- 泵站下游10kV_50km/LConn2
  Three-Phase V-I Measurement3/RConn3 -- 泵站上游10kV_20km/LConn3 -- 泵站下游10kV_50km/LConn3
  泵站下游综合 等效负载40KW/LConn1 -- 泵站下游10kV_50km/RConn1
  泵站下游综合 等效负载40KW/LConn2 -- 泵站下游10kV_50km/RConn2
  泵站下游综合 等效负载40KW/LConn3 -- 泵站下游10kV_50km/RConn3
  泵站上游综合 等效负载20KW/LConn1 -- 泵站上游10kV_20km/RConn1
  泵站上游综合 等效负载20KW/LConn2 -- 泵站上游10kV_20km/RConn2
  泵站上游综合 等效负载20KW/LConn3 -- 泵站上游10kV_20km/RConn3
  等效线路1 100m/LConn1 -- Three-Phase V-I Measurement1/RConn1
  等效线路 100m1/LConn1 -- Three-Phase V-I Measurement1/RConn2
  等效线路 100m2/LConn1 -- Three-Phase V-I Measurement1/RConn3
  IT_Transformer 400/400 星方式250kVA/LConn1 -- IT_Transformer 400/230 相方式30kVA/LConn1 -- "    厂房TN系统 等效负载 单相10kw1"/LConn1 -- A相接地 0.4-0.5s/LConn1 -- 等效线路 100m6/LConn1 -- 等效线路 100m5/LConn1 -- 等效线路1 100m/RConn1
  IT_Transformer 400/400 星方式250kVA/LConn2 -- IT_Transformer 400/230 相方式30kVA/LConn2 -- "    厂房TN系统 等效负载 单相30kw"/LConn1 -- A相接地 0.4-0.5s/LConn2 -- 等效线路 100m3/LConn1 -- 等效线路 100m4/LConn1 -- 等效线路 100m1/RConn1
  IT_Transformer 400/400 星方式250kVA/LConn3 -- IT_Transformer 400/230 相方式30kVA/LConn3 -- Series RLC Load8/LConn1 -- A相接地 0.4-0.5s/LConn3 -- 等效线路1 100m2/LConn1 -- 等效线路1 100m1/LConn1 -- 等效线路 100m2/RConn1
  线路1 100m/LConn2 -- 线路3 100m/LConn2 -- 线路4 100m/LConn2 -- 线路2 100m/LConn2 -- Three-Phase V-I Measurement6/RConn2
  线路1 100m/LConn1 -- 线路3 100m/LConn1 -- 线路4 100m/LConn1 -- 线路2 100m/LConn1 -- Three-Phase V-I Measurement6/RConn1
  Three-Phase V-I Measurement6/RConn3 -- 线路2 100m/LConn3 -- 线路3 100m/LConn3 -- 线路4 100m/LConn3 -- 线路1 100m/LConn3
  1#机组/LConn1 -- 线路1 100m/RConn1
  1#机组/LConn2 -- 线路1 100m/RConn2
  1#机组/LConn3 -- 线路1 100m/RConn3
  2#机组/LConn1 -- 线路2 100m/RConn1
  2#机组/LConn2 -- 线路2 100m/RConn2
  2#机组/LConn3 -- 线路2 100m/RConn3
  线路4 100m/RConn1 -- 4#机组/LConn1
  线路4 100m/RConn2 -- 4#机组/LConn2
  线路4 100m/RConn3 -- 4#机组/LConn3
  5#机组/LConn3 -- 线路5 100m/RConn3
  5#机组/LConn1 -- 线路5 100m/RConn1
  5#机组/LConn2 -- 线路5 100m/RConn2
  6#机组/LConn3 -- 线路6 100m/RConn3
  6#机组/LConn2 -- 线路6 100m/RConn2
  6#机组/LConn1 -- 线路6 100m/RConn1
  增容机组/LConn1 -- 增容 线路/RConn1
  增容机组/LConn2 -- 增容 线路/RConn2
  增容机组/LConn3 -- 增容 线路/RConn3
  线路3 100m/RConn1 -- 3#机组/LConn1
  线路3 100m/RConn2 -- 3#机组/LConn2
  线路3 100m/RConn3 -- 3#机组/LConn3
  7#机组/LConn3 -- 线路7 100m/RConn3
  7#机组/LConn2 -- 线路7 100m/RConn2
  7#机组/LConn1 -- 线路7 100m/RConn1
  高阻抗 接地20kΩ/RConn1 -- Ground3/LConn1 -- Voltage Measurement1/LConn2
  Series RLC Load2/LConn1 -- 技术供水 电机380V 5.5kw 1#/LConn1 -- 其他三相 设备等效 55kw/LConn1 -- B相接地 0.2-0.3s/LConn1 -- A相接地 0.1-0.3s/LConn1 -- Three-Phase V-I Measurement4/RConn1 -- Voltage Measurement/LConn1
  Series RLC Load1/LConn1 -- 其他三相 设备等效 55kw/LConn2 -- 技术供水 电机380V 5.5kw 1#/LConn2 -- B相接地 0.2-0.3s/LConn2 -- A相接地 0.1-0.3s/LConn2 -- Three-Phase V-I Measurement4/RConn2
  星方式 下220V 等效负 载10kw/LConn1 -- Three-Phase V-I Measurement4/RConn3 -- Voltage Measurement2/LConn1 -- 技术供水 电机380V 5.5kw 1#/LConn3 -- B相接地 0.2-0.3s/LConn3 -- A相接地 0.1-0.3s/LConn3 -- 其他三相 设备等效 55kw/LConn3
  Series RLC Load2/RConn1 -- Series RLC Load1/RConn1 -- 星方式 下220V 等效负 载10kw/RConn1 -- Voltage Measurement1/LConn1 -- 高阻抗 接地20kΩ/LConn1 -- IT_Transformer 400/400 星方式250kVA/RConn4 -- Voltage Measurement2/LConn2 -- Voltage Measurement/LConn2
  IT_Transformer 400/400 星方式250kVA/RConn3 -- Three-Phase V-I Measurement4/LConn3
  IT_Transformer 400/400 星方式250kVA/RConn2 -- Three-Phase V-I Measurement4/LConn2
  IT_Transformer 400/400 星方式250kVA/RConn1 -- Three-Phase V-I Measurement4/LConn1
  Series RLC Load3/LConn1 -- Three-Phase PI Section Line/RConn1 -- 相方式下 220V等效 负载10kw/LConn1
  Series RLC Load3/RConn1 -- Three-Phase PI Section Line/RConn2 -- Series RLC Load4/LConn1
  相方式下 220V等效 负载10kw/RConn1 -- Series RLC Load4/RConn1 -- Three-Phase PI Section Line/RConn3
  IT_Transformer 400/230 相方式30kVA/RConn1 -- Three-Phase V-I Measurement7/LConn1
  IT_Transformer 400/230 相方式30kVA/RConn2 -- Three-Phase V-I Measurement7/LConn2
  IT_Transformer 400/230 相方式30kVA/RConn3 -- Three-Phase V-I Measurement7/LConn3
  41B所变 35/0.4_500kVA/RConn4 -- Ground1/LConn1 -- 到厂房 线路 100m/LConn1
  Series RLC Load6/LConn1 -- 等效线路 100m5/RConn1
  Series RLC Load5/LConn1 -- 等效线路 100m4/RConn1
  南办公楼 等效负载 每相10kw/LConn1 -- 等效线路1 100m1/RConn1
  到厂房 线路 100m/RConn1 -- 北楼线路 200m/LConn1 -- Series RLC Load8/RConn1 -- "    厂房TN系统 等效负载 单相10kw1"/RConn1 -- "    厂房TN系统 等效负载 单相30kw"/RConn1 -- 南楼线路 100m/LConn1
  南楼线路 100m/RConn1 -- Series RLC Load6/RConn1 -- Series RLC Load5/RConn1 -- 南办公楼 等效负载 每相10kw/RConn1
  Series RLC Load9/LConn1 -- 等效线路 100m6/RConn1
  Series RLC Load7/LConn1 -- 等效线路 100m3/RConn1
  北办公楼 等效负载 每相20kw/LConn1 -- 等效线路1 100m2/RConn1
  北楼线路 200m/RConn1 -- Series RLC Load9/RConn1 -- Series RLC Load7/RConn1 -- 北办公楼 等效负载 每相20kw/RConn1
  Three-Phase PI Section Line/LConn3 -- Three-Phase V-I Measurement7/RConn3
  Three-Phase PI Section Line/LConn2 -- Three-Phase V-I Measurement7/RConn2
  Three-Phase PI Section Line/LConn1 -- Three-Phase V-I Measurement7/RConn1
